simulink model "Adp_Lgt_SytmV2"  (R2021a)
settings: Solver=FixedStepDiscrete  StartTime=0.0  StopTime=1149  FixedStep=1  RelTol=1e-3
libraries: simulink x7
(part 2 of 2)

== stateflow chart Adp_Lgt_SytmV2/Adp_Lgt_Subsystem/Adp_Lgt_Enabled_Subsystem/Adp_Lgt_Enabled_Subsystem1/Adp_Lgt_Subsystem1/Adp_Lgt_Enabled Subsystem1/Highway/Detect_Object_Enable_Subsystem/Chart ==
  state Initial_Beam_Condition
    Low_Beam1=0;
    High_Beam1=1;
  state Object_Detect_In_Lane1 [group]
    state PedestrainOrAnimal_DetectedL1
      Low_Beam1=1;
      High_Beam1=0;
    state CyclistOrMCyclistOrTWheeler
      Low_Beam1=1;
      High_Beam1=0;
    state CarOrMiniBusOrLCV
      Low_Beam1=1;
      High_Beam1=0;
    state BusOrTruck
      Low_Beam1=1;
      High_Beam1=0;
    (junction 3) -> PedestrainOrAnimal_DetectedL1 [order 1] : [(Detect_Object==1) && (Long_Dist<= 25)]
    PedestrainOrAnimal_DetectedL1 -> (junction 23) : [(Long_Dist<=5) || (Detect_Object~=1)]
    (junction 3) -> (junction 10) [order 2]
    (junction 23) -> (junction 26)
    (junction 10) -> Object_Detect_In_Lane1.CyclistOrMCyclistOrTWheeler [order 1] : [(Detect_Object==2) && (Long_Dist<=50)]
    Object_Detect_In_Lane1.CyclistOrMCyclistOrTWheeler -> (junction 26) : [(Long_Dist<=5) || (Detect_Object~=2)]
    (junction 10) -> (junction 16) [order 2]
    (junction 26) -> (junction 29)
    (junction 16) -> Object_Detect_In_Lane1.CarOrMiniBusOrLCV [order 1] : [(Detect_Object==3) && (Long_Dist<=75)]
    Object_Detect_In_Lane1.CarOrMiniBusOrLCV -> (junction 29) : [(Long_Dist<=5) || (Detect_Object~=3)]
    (junction 16) -> (junction 19) [order 2]
    (junction 29) -> (junction 33)
    (junction 19) -> Object_Detect_In_Lane1.BusOrTruck [order 1] : [(Detect_Object==4) && (Long_Dist<=100)]
    Object_Detect_In_Lane1.BusOrTruck -> (junction 33) : [(Long_Dist<=5) || (Detect_Object~=4)]
    (junction 19) -> (junction 40) [order 2]
    (junction 33) -> (junction 38)
    (junction 38) -> (junction 40)
  state Object_Detect_In_Lane2 [group]
    state PedestrainOrAnimal_Detected
      Low_Beam1=1;
      High_Beam1=0;
    state CyclistOrMCyclistOrTWheeler
      Low_Beam1=1;
      High_Beam1=0;
    state CarOrMiniBusOrLCV
      Low_Beam1=1;
      High_Beam1=0;
    state BusOrTruck
      Low_Beam1=1;
      High_Beam1=0;
    (junction 44) -> Object_Detect_In_Lane2.PedestrainOrAnimal_Detected [order 1] : [(Detect_Object==1) && (Long_Dist<=30)]
    Object_Detect_In_Lane2.PedestrainOrAnimal_Detected -> (junction 57) : [(Long_Dist<=10) || (Detect_Object~=1)]
    (junction 44) -> (junction 59) [order 2]
    (junction 57) -> (junction 60)
    (junction 59) -> Object_Detect_In_Lane2.CyclistOrMCyclistOrTWheeler [order 1] : [(Detect_Object==2) && (Long_Dist<=55)]
    Object_Detect_In_Lane2.CyclistOrMCyclistOrTWheeler -> (junction 60) : [(Long_Dist<=10) || (Detect_Object~=2)]
    (junction 59) -> (junction 62) [order 2]
    (junction 60) -> (junction 56)
    (junction 62) -> Object_Detect_In_Lane2.CarOrMiniBusOrLCV [order 1] : [(Detect_Object==3) && (Long_Dist<=80)]
    Object_Detect_In_Lane2.CarOrMiniBusOrLCV -> (junction 56) : [(Long_Dist<=10) || (Detect_Object~=3)]
    (junction 62) -> (junction 64) [order 2]
    (junction 56) -> (junction 50)
    (junction 64) -> Object_Detect_In_Lane2.BusOrTruck [order 1] : [(Detect_Object==4) && (Long_Dist<=105)]
    Object_Detect_In_Lane2.BusOrTruck -> (junction 50) : [(Long_Dist<=10) || (Detect_Object~=4)]
    (junction 64) -> (junction 51) [order 2]
    (junction 50) -> (junction 65)
    (junction 65) -> (junction 51)
  state Object_Detect_In_Lane3 [group]
    state PedestrainOrAnimal_Detected
      Low_Beam1=1;
      High_Beam1=0;
    state CyclistOrMCyclistOrTWheeler
      Low_Beam1=1;
      High_Beam1=0;
    state CarOrMiniBusOrLCV
      Low_Beam1=1;
      High_Beam1=0;
    state BusOrTruck
      Low_Beam1=1;
      High_Beam1=0;
    (junction 116) -> Object_Detect_In_Lane3.PedestrainOrAnimal_Detected [order 1] : [(Detect_Object==1) && (Long_Dist<= 35)]
    Object_Detect_In_Lane3.PedestrainOrAnimal_Detected -> (junction 129) : [(Long_Dist<=15) || (Detect_Object~=1)]
    (junction 116) -> (junction 131) [order 2]
    (junction 129) -> (junction 132)
    (junction 131) -> Object_Detect_In_Lane3.CyclistOrMCyclistOrTWheeler [order 1] : [(Detect_Object==2) && (Long_Dist<=60)]
    Object_Detect_In_Lane3.CyclistOrMCyclistOrTWheeler -> (junction 132) : [(Long_Dist<=15) || (Detect_Object~=2)]
    (junction 131) -> (junction 134) [order 2]
    (junction 132) -> (junction 128)
    (junction 134) -> Object_Detect_In_Lane3.CarOrMiniBusOrLCV [order 1] : [(Detect_Object==3) && (Long_Dist<=85)]
    Object_Detect_In_Lane3.CarOrMiniBusOrLCV -> (junction 128) : [(Long_Dist<=15) || (Detect_Object~=3)]
    (junction 134) -> (junction 136) [order 2]
    (junction 128) -> (junction 122)
    (junction 136) -> Object_Detect_In_Lane3.BusOrTruck [order 1] : [(Detect_Object==4) && (Long_Dist<=110)]
    Object_Detect_In_Lane3.BusOrTruck -> (junction 122) : [(Long_Dist<=15) || (Detect_Object~=4)]
    (junction 136) -> (junction 123) [order 2]
    (junction 122) -> (junction 137)
    (junction 137) -> (junction 123)
  state Object_Detect_In_Lane4 [group]
    state PedestrainOrAnimal_Detected
      Low_Beam1=1;
      High_Beam1=0;
    state CyclistOrMCyclistOrTWheeler
      Low_Beam1=1;
      High_Beam1=0;
    state CarOrMiniBusOrLCV
      Low_Beam1=1;
      High_Beam1=0;
    state BusOrTruck
      Low_Beam1=1;
      High_Beam1=0;
    (junction 164) -> Object_Detect_In_Lane4.PedestrainOrAnimal_Detected [order 1] : [(Detect_Object==1) && (Long_Dist<= 40)]
    Object_Detect_In_Lane4.PedestrainOrAnimal_Detected -> (junction 168) : [(Long_Dist<=20) || (Detect_Object~=1)]
    (junction 164) -> (junction 170) [order 2]
    (junction 168) -> (junction 160)
    (junction 170) -> Object_Detect_In_Lane4.CyclistOrMCyclistOrTWheeler [order 1] : [(Detect_Object==2) && (Long_Dist<=65)]
    Object_Detect_In_Lane4.CyclistOrMCyclistOrTWheeler -> (junction 160) : [(Long_Dist<=20) || (Detect_Object~=2)]
    (junction 170) -> (junction 172) [order 2]
    (junction 160) -> (junction 166)
    (junction 172) -> Object_Detect_In_Lane4.CarOrMiniBusOrLCV [order 1] : [(Detect_Object==3) && (Long_Dist<=90)]
    Object_Detect_In_Lane4.CarOrMiniBusOrLCV -> (junction 166) : [(Long_Dist<=20) || (Detect_Object~=3)]
    (junction 172) -> (junction 167) [order 2]
    (junction 166) -> (junction 169)
    (junction 167) -> Object_Detect_In_Lane4.BusOrTruck [order 1] : [(Detect_Object==4) && (Long_Dist<=115)]
    Object_Detect_In_Lane4.BusOrTruck -> (junction 169) : [(Long_Dist<=20) || (Detect_Object~=4)]
    (junction 167) -> (junction 174) [order 2]
    (junction 169) -> (junction 157)
    (junction 157) -> (junction 174)
  state Object_Detect_In_Lane5 [group]
    state PedestrainOrAnimal_Detected
      Low_Beam1=1;
      High_Beam1=0;
    state CyclistOrMCyclistOrTWheeler
      Low_Beam1=1;
      High_Beam1=0;
    state CarOrMiniBusOrLCV
      Low_Beam1=1;
      High_Beam1=0;
    state BusOrTruck
      Low_Beam1=1;
      High_Beam1=0;
    (junction 229) -> Object_Detect_In_Lane5.PedestrainOrAnimal_Detected [order 1] : [(Detect_Object==1) && (Long_Dist<= 45)]
    Object_Detect_In_Lane5.PedestrainOrAnimal_Detected -> (junction 230) : [(Long_Dist<=25) || (Detect_Object~=1)]
    (junction 229) -> (junction 233) [order 2]
    (junction 230) -> (junction 235)
    (junction 233) -> Object_Detect_In_Lane5.CyclistOrMCyclistOrTWheeler [order 1] : [(Detect_Object==2) && (Long_Dist<=70)]
    Object_Detect_In_Lane5.CyclistOrMCyclistOrTWheeler -> (junction 235) : [(Long_Dist<=25) || (Detect_Object~=2)]
    (junction 233) -> (junction 236) [order 2]
    (junction 235) -> (junction 220)
    (junction 236) -> Object_Detect_In_Lane5.CarOrMiniBusOrLCV [order 1] : [(Detect_Object==3) && (Long_Dist<=95)]
    Object_Detect_In_Lane5.CarOrMiniBusOrLCV -> (junction 220) : [(Long_Dist<=25) || (Detect_Object~=3)]
    (junction 236) -> (junction 231) [order 2]
    (junction 220) -> (junction 221)
    (junction 231) -> Object_Detect_In_Lane5.BusOrTruck [order 1] : [(Detect_Object==4) && (Long_Dist<=120)]
    Object_Detect_In_Lane5.BusOrTruck -> (junction 221) : [(Long_Dist<=25) || (Detect_Object~=4)]
    (junction 231) -> (junction 234) [order 2]
    (junction 221) -> (junction 237)
    (junction 237) -> (junction 234)
  (default) -> Initial_Beam_Condition
  Initial_Beam_Condition -> (junction 3) [order 1] : [Left_Lane==1]
  (junction 40) -> Initial_Beam_Condition
  Initial_Beam_Condition -> (junction 44) [order 2] : [Left_Lane==2]
  (junction 51) -> Initial_Beam_Condition
  Initial_Beam_Condition -> (junction 116) [order 3] : [Left_Lane==3]
  (junction 123) -> Initial_Beam_Condition
  Initial_Beam_Condition -> (junction 164) [order 4] : [Left_Lane==4]
  (junction 174) -> Initial_Beam_Condition
  Initial_Beam_Condition -> (junction 229) [order 5] : [Left_Lane==5]
  (junction 234) -> Initial_Beam_Condition
  data: Left_Lane input uint8; Long_Dist input uint8; High_Beam1 output int8; Low_Beam1 output int8; Detect_Object input uint8

== stateflow chart Adp_Lgt_SytmV2/Adp_Lgt_Subsystem/Adp_Lgt_Enabled_Subsystem/Adp_Lgt_Enabled_Subsystem1/Adp_Lgt_Subsystem1/Adp_Lgt_Enabled Subsystem1/Highway/Lane_Detection/Chart ==
  state Initial_Beam_Condition
    Left_Lane=0;
  state Lane_1
    Left_Lane=1;
  state Lane_2
    Left_Lane=2;
  state Lane_3
    Left_Lane=3;
  state Lane_4
    Left_Lane=4;
  state Lane_5
    Left_Lane=5;
  (default) -> Initial_Beam_Condition
  Initial_Beam_Condition -> Lane_1 [order 2] : [((Long_Dist<=150) && (LateralDistance>1 && LateralDistance<=4.7))]
  Lane_1 -> Initial_Beam_Condition : [Long_Dist<=5]
  Initial_Beam_Condition -> Lane_2 [order 3] : [((Long_Dist<=150) && (LateralDistance>4.8 && LateralDistance<=8.5))]
  Lane_2 -> Initial_Beam_Condition : [Long_Dist<=10]
  Initial_Beam_Condition -> Lane_3 [order 5] : [((Long_Dist<=150) && (LateralDistance>8.6 && LateralDistance<=12.3))]
  Lane_3 -> Initial_Beam_Condition : [Long_Dist<=15]
  Initial_Beam_Condition -> Lane_4 [order 4] : [((Long_Dist<=150) && (LateralDistance>12.4 && LateralDistance<=16.1))]
  Lane_4 -> Initial_Beam_Condition : [Long_Dist<=20]
  Initial_Beam_Condition -> Lane_5 [order 1] : [((Long_Dist<=150) && (LateralDistance>16.2 && LateralDistance<=19.9))]
  Lane_5 -> Initial_Beam_Condition : [Long_Dist<=25]
  data: Left_Lane output uint8; LateralDistance input double; Long_Dist input uint8

== stateflow chart Adp_Lgt_SytmV2/Adp_Lgt_Subsystem/Adp_Lgt_Enabled_Subsystem/Adp_Lgt_Enabled_Subsystem1/Adp_Lgt_Subsystem1/Adp_Lgt_Enabled Subsystem1/UPHILL_AND_DOWNHILL/Chart ==
  settings: updateMethod=DISCRETE  sampleTime=1
  state Downhill_beam_setting1
    High_Beam2=0;
    Low_Beam2=1;
    Servo_Motr=1;
    Beam_Agl_Setting=3;
    Tilt_angle=Gyro_Angle+2;
  state On_Delay1
    en:
    i=0;
    du:
    i=i+y;
  state On_Delay
    en:
    i=0;
    du:
    i=i+y;
  state Uphill_beam_setting1
    High_Beam2=0;
    Low_Beam2=1;
    Servo_Motr=1;
    Beam_Agl_Setting=2;
    Tilt_angle=Gyro_Angle-2;
  state Default_beam_setting
    High_Beam2=1;
    Low_Beam2=0;
    Servo_Motr=0;
    Beam_Agl_Setting=0;
    Tilt_angle=Gyro_Angle;
  state Uphill_beam_setting2
    High_Beam2=0;
    Low_Beam2=1;
    Servo_Motr=1;
    Beam_Agl_Setting=2;
    Tilt_angle=Gyro_Angle-4;
  state Downhill_beam_setting2
    High_Beam2=0;
    Low_Beam2=1;
    Servo_Motr=1;
    Beam_Agl_Setting=4;
    Tilt_angle=Gyro_Angle+4;
  state On_Delay3
    en:
    i=0;
    du:
    i=i+y;
  state On_Delay2
    en:
    i=0;
    du:
    i=i+y;
  (default) -> Default_beam_setting
  (junction 121) -> Downhill_beam_setting1 [order 1] : [(Speed<=40)&&(Gyro_Angle<-5)]
  On_Delay1 -> (junction 121) : [i>=Time_Step]
  On_Delay -> (junction 111) : [i>=Time_Step]
  (junction 111) -> Uphill_beam_setting1 [order 1] : [(Speed<=40)&&(Gyro_Angle>5)]
  Default_beam_setting -> On_Delay1 [order 4] : [Gyro_Angle<-5&&Gyro_Angle>=-10]
  Default_beam_setting -> On_Delay [order 1] : [(Gyro_Angle>5&&Gyro_Angle<=10)]
  (junction 121) -> (junction 123) [order 2]
  (junction 111) -> (junction 115) [order 2]
  Downhill_beam_setting1 -> (junction 123) [order 1] : after(3,sec)[Gyro_Angle>=-5]
  (junction 123) -> Default_beam_setting
  (junction 115) -> Default_beam_setting
  Uphill_beam_setting1 -> (junction 115) [order 2] : after(3,sec)[Gyro_Angle<=5]
  Downhill_beam_setting1 -> On_Delay3 [order 2] : [(Gyro_Angle<-10)||(Speed>40)]
  (junction 59) -> Downhill_beam_setting1
  (junction 20) -> Uphill_beam_setting1
  Uphill_beam_setting1 -> On_Delay2 [order 1] : [(Gyro_Angle>10)||(Speed>40)]
  Uphill_beam_setting2 -> Default_beam_setting [order 2] : [(Speed<40)&&(Gyro_Angle<=5)]
  Uphill_beam_setting2 -> (junction 20) [order 1] : after(3,sec)[(Speed<40)&&(Gyro_Angle<=10&&Gyro_Angle>5)]
  Downhill_beam_setting2 -> Default_beam_setting [order 2] : [(Speed<40)&&(Gyro_Angle>=-5)]
  (junction 118) -> (junction 20) [order 2]
  Downhill_beam_setting2 -> (junction 59) [order 1] : after(3,sec)[(Speed<40)&&(Gyro_Angle>=-10)]
  (junction 126) -> (junction 59) [order 2]
  Default_beam_setting -> Downhill_beam_setting2 [order 3] : [(Speed>40)&&(Gyro_Angle<-5)]
  Default_beam_setting -> Uphill_beam_setting2 [order 2] : [(Speed>40)&&(Gyro_Angle>5)]
  (junction 118) -> Uphill_beam_setting2 [order 1] : [(Gyro_Angle>10)||(Speed>40)]
  On_Delay2 -> (junction 118) : [i>=Time_Step]
  On_Delay3 -> (junction 126) : [i>=Time_Step]
  (junction 126) -> Downhill_beam_setting2 [order 1] : [(Gyro_Angle<-10)||(Speed>40)]
  data: Gyro_Angle input int8; Speed input uint8; Time_Step input; High_Beam2 output int8; Low_Beam2 output int8; i local; y constant double [0..1] =1; Beam_Agl_Setting local; Servo_Motr local; Tilt_angle local

== stateflow chart Adp_Lgt_SytmV2/Adp_Lgt_Subsystem/Adp_Lgt_Enabled_Subsystem/Adp_Lgt_Enabled_Subsystem1/Adp_Lgt_Subsystem1/Foglight_System/Fog_Light/Chart ==
  settings: updateMethod=DISCRETE  sampleTime=1  initializeOutput=1
  state NoFog
    High_Beam4=1;
    Low_Beam4=0;
    FogLight=0;
    HazardLight=0;
  state ModrateFog
    High_Beam4=0;
    Low_Beam4=1;
    FogLight=1;
    HazardLight=0;
  state LightFog
    High_Beam4=0;
    Low_Beam4=1;
    FogLight=0;
    HazardLight=0;
  state HeayFog
    High_Beam4=0;
    Low_Beam4=1;
    FogLight=1;
    HazardLight=1;
  (default) -> NoFog
  NoFog -> (junction 112) : [Fog~=0]
  (junction 151) -> NoFog : [Fog==0]
  ModrateFog -> (junction 127) : [Fog~=2]
  (junction 127) -> (junction 112)
  (junction 112) -> (junction 151) [order 4]
  (junction 112) -> ModrateFog [order 2] : [Fog==2]
  (junction 112) -> LightFog [order 1] : [Fog==1]
  (junction 134) -> (junction 112)
  (junction 146) -> (junction 112)
  (junction 112) -> HeayFog [order 3] : [Fog==3]
  LightFog -> (junction 134) : [Fog~=1]
  HeayFog -> (junction 146) : [Fog~=3]
  data: Fog input uint8; FogLight output =0; HazardLight output =0; High_Beam4 output int8 =0; Low_Beam4 output int8 =0

== stateflow chart Adp_Lgt_SytmV2/Adp_Lgt_Subsystem/Adp_Lgt_Enabled_Subsystem/Adp_Lgt_Enabled_Subsystem1/Adp_Lgt_Subsystem1/Foglight_System/Wiper_Detection/Chart ==
  state Delay
    en:
    temp=0;
    du:
    temp=temp+1;
  state WiperONOff
    High_Beam5=0;
    Low_Beam5=1;
    ex:
    High_Beam5=0;
    Low_Beam5=0;
  state Defalult
  (default) -> Defalult
  Delay -> WiperONOff [order 1] : [temp>=120]
  Defalult -> Delay : [Wiper==1]
  Delay -> Defalult [order 2] : [Wiper==0]
  WiperONOff -> Delay : [Wiper==0]
  data: Wiper input; temp local; High_Beam5 output int8; Low_Beam5 output int8

== stateflow chart Adp_Lgt_SytmV2/Adp_Lgt_Subsystem/Adp_Lgt_Enabled_Subsystem/Adp_Lgt_Enabled_Subsystem1/Ambiant_Light/Chart ==
  settings: updateMethod=DISCRETE  sampleTime=1
  state AmbientLedLight_ON
    LedLight=1;
  state AmbientLedLight_OFF
    LedLight=0;
  (default) -> AmbientLedLight_OFF
  AmbientLedLight_OFF -> AmbientLedLight_ON : [Lightswitch==1]
  AmbientLedLight_ON -> AmbientLedLight_OFF [order 1] : [duration (ignitionon==1&&Lightswitch==0)>20]
  AmbientLedLight_ON -> AmbientLedLight_OFF [order 2] : [Lock==1]
  data: ignitionon input boolean; Lock input; Lightswitch input boolean; LedLight output int8

== stateflow chart Adp_Lgt_SytmV2/Adp_Lgt_Subsystem/Adp_Lgt_Enabled_Subsystem/Adp_Lgt_Enabled_Subsystem1/Default_Beam_Enable_Subsytem/Chart ==
  settings: updateMethod=DISCRETE  sampleTime=1
  state Default_Beam_Mode
    en:
    High_Beam_Defualt=0;
    Low_Beam_Defualt=1;
  (default) -> Default_Beam_Mode
  data: High_Beam_Defualt output int8; Low_Beam_Defualt output int8

== stateflow chart Adp_Lgt_SytmV2/Adp_Lgt_Subsystem/Adp_Lgt_Enabled_Subsystem/Exterior_Light_Subsystem/Chart ==
  state Light
    state ExtreiorLight
      state FRHSIndicator [parallel]
        FRHSIndicator=1;
        settings: executionOrder=1
      state FLHSIndicator [parallel]
        FLHSIndicator=1;
        settings: executionOrder=2
      state BLHSindicator [parallel]
        BLHSIndicator=1
        settings: executionOrder=3
      state BRHSIndicator [parallel]
        BRHSIndicator=1
        settings: executionOrder=4
      state LHS_FrontLight [parallel]
        settings: executionOrder=5
      state RHS_FronLightt [parallel]
        settings: executionOrder=6
    (default) -> ExtreiorLight : {Exterior_Light=1
        | HLHSIndicator=1
        | HRHSIndicator=1}
  state DashBoard
    Exterior_Light=0
    FLHSIndicator=0
    FRHSIndicator=0
    BLHSIndicator=0
    BRHSIndicator=0
    HLHSIndicator=0
    HRHSIndicator=0
  (default) -> DashBoard
  DashBoard -> Light : [(Key==0&&ignitionon==0)]
  Light -> DashBoard : after(5,sec)
  data: Key input boolean; Exterior_Light output int8; FRHSIndicator output int8; BLHSIndicator output int8; HRHSIndicator output int8; BRHSIndicator output int8; HLHSIndicator output int8; FLHSIndicator output int8; ignitionon input
